simulink model "General_Stablised_Power_R2020a"  (R2020a)
settings: Solver=VariableStepAuto  StartTime=0.0  StopTime=10.0  FixedStep=1e-12  RelTol=1e-3
values from neighbouring files (symbols this model uses):
  Torque_Load = 1    [Parameters.m]
libraries: fl_lib x18, nesl_utility x18, ee_lib x13
settings Model: Creator=YXL1108  LastModifiedBy=YXL1108
settings SolverCC: ZeroCrossAlgorithm=Adaptive
settings DebuggingCC: IgnoredZcDiagnostic=none

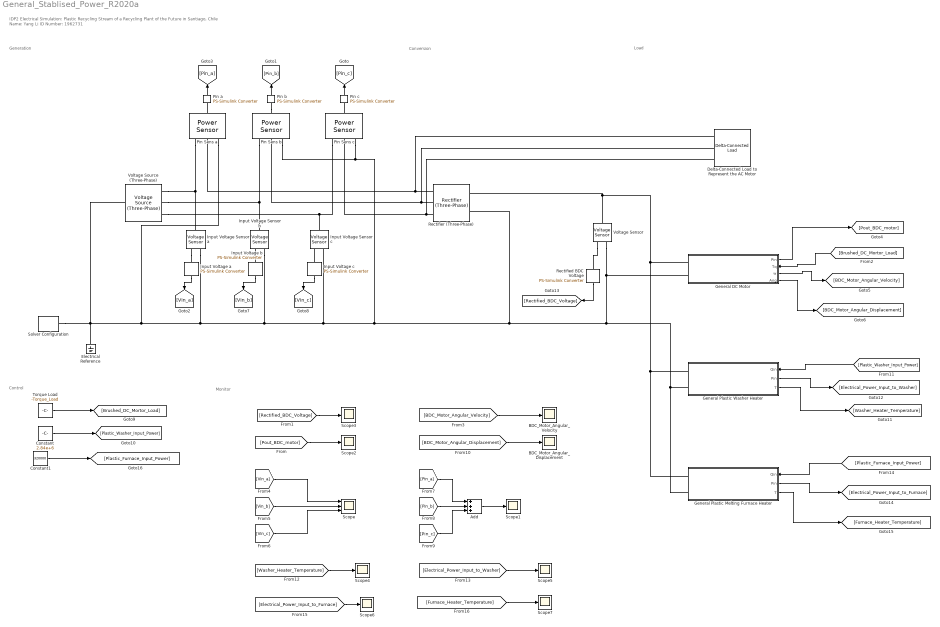
== system General_Stablised_Power_R2020a ==
  note: Control
  note: Load
  note: Conversion
  note: Monitor
  note: Generation
  note: IDP2 Electrical Simulation: Plastic Recycling Stream of a Recycling Plant of the Future in Santiago, Chile
      | Name: Yang Li
      | ID Number: 1962731
  Add : Sum  Inputs=+++
  BDC_Motor_Angular_Displacement : Scope
  BDC_Motor_Angular_Velocity : Scope
  Constant : Constant  Value=2.84e+6
  Constant1 : Constant  Value=320000
  Delta-Connected Load to Represent the AC Motor : ee_lib/Passive/RLC Assemblies/Delta-Connected Load  parameterization=2  component_structure=1  component_structure_PQ=4  R=1 Ohm  L=1e-3 H  C=1e-6 F  IL0=[0, 0, 0] A  VC0=[0, 0, 0] V  R_parasitic=1e-6 Ohm  G_parasitic=1e-6 1/Ohm  VRated=380 V  FRated=50 Hz  P=45 kW  Qpos=1e2 V*A  Qneg=-1e2 V*A  Vmag0=380 V  Vang0=0 deg  Freq0=50 Hz  R_parasitic_PQ=1e-6 Ohm  G_parasitic_PQ=1e-6 1/Ohm
      settings: SourceProductBaseCode=PS  InternalSimscapePortConfiguration="{\"Bottom\":[],\"Left\":[{\"id\":\"a\",\"label\":\"a\",\"type\":\"foundation.electrical.electrical\"},{\"id\":\"b\",\"label\":\"b\",\"type\":\"foundation.electrical.electrical\"},{\"id\":\"c\",\"label\":\"c\",\"type\":\"foundation.electrical.electrical\"}],\"Right\":[],\"Top\":[]}"
  Electrical Reference : fl_lib/Electrical/Electrical Elements/Electrical Reference
  General DC Motor : Subsystem
      settings: PortSchema="{\"entries\":[{\"content\":{\"sides\":[{\"content\":{\"connectorIds\":[\"LConn1\",\"LConn2\"]},\"type\":\"ConnectorPlacement.EquallySpacedRectSide\",\"uuid\":\"f4c4afdb-1f07-4496-beab-7bd7d7d73664\"},{\"content\":{\"connectorIds\":[\"Out1\",\"In1\",\"Out2\",\"Out3\"],\"side\":\"RIGHT\"},\"type\":\"ConnectorPlacement.EquallySpacedRectSide\",\"uuid\":\"dc37d443-6c2c-49b1-8221-5c741536e800\"},{\"content\":{\"connectorIds\":[],\"side\":\"TOP\"},\"type\":\"ConnectorPlacement.EquallySpacedRectSide\",\"uuid\":\"4c68adcc-5338-4c92-85dc-69672cfb0c08\"}]},\"type\":\"ConnectorPlacement.EquallySpacedConnector\",\"uuid\":\"b4ec0e54-21aa-4bd3-95d2-2023b489fb55\"}],\"packageUris\":[\"http://schema.mathworks.com/mf0/Connector/19700101\"],\"version\":\"1.0\"}"
  General Plastic Melting Furnace Heater : Subsystem
      settings: PortSchema="{\"entries\":[{\"content\":{\"sides\":[{\"content\":{\"connectorIds\":[\"LConn1\",\"LConn2\"]},\"type\":\"ConnectorPlacement.EquallySpacedRectSide\",\"uuid\":\"1fa59fc7-be06-49d0-a9b5-9f39dbd9f596\"},{\"content\":{\"connectorIds\":[\"In1\",\"Out1\",\"Out2\"],\"side\":\"RIGHT\"},\"type\":\"ConnectorPlacement.EquallySpacedRectSide\",\"uuid\":\"e02b180c-81d7-4bb9-9dca-301601ef73bf\"},{\"content\":{\"connectorIds\":[],\"side\":\"TOP\"},\"type\":\"ConnectorPlacement.EquallySpacedRectSide\",\"uuid\":\"9bedab00-a6ba-4834-a03a-1eed8c48595a\"}]},\"type\":\"ConnectorPlacement.EquallySpacedConnector\",\"uuid\":\"acdf9e6b-b46a-43ad-9e2b-2b45ab9d2f8b\"}],\"packageUris\":[\"http://schema.mathworks.com/mf0/Connector/19700101\"],\"version\":\"1.0\"}"
  General Plastic Washer Heater : Subsystem
      settings: PortSchema="{\"entries\":[{\"content\":{\"sides\":[{\"content\":{\"connectorIds\":[\"LConn1\",\"LConn2\"]},\"type\":\"ConnectorPlacement.EquallySpacedRectSide\",\"uuid\":\"1fa59fc7-be06-49d0-a9b5-9f39dbd9f596\"},{\"content\":{\"connectorIds\":[\"In1\",\"Out1\",\"Out2\"],\"side\":\"RIGHT\"},\"type\":\"ConnectorPlacement.EquallySpacedRectSide\",\"uuid\":\"e02b180c-81d7-4bb9-9dca-301601ef73bf\"},{\"content\":{\"connectorIds\":[],\"side\":\"TOP\"},\"type\":\"ConnectorPlacement.EquallySpacedRectSide\",\"uuid\":\"9bedab00-a6ba-4834-a03a-1eed8c48595a\"}]},\"type\":\"ConnectorPlacement.EquallySpacedConnector\",\"uuid\":\"acdf9e6b-b46a-43ad-9e2b-2b45ab9d2f8b\"}],\"packageUris\":[\"http://schema.mathworks.com/mf0/Connector/19700101\"],\"version\":\"1.0\"}"
  Input Voltage Sensor a : fl_lib/Electrical/Electrical Sensors/Voltage Sensor
  Input Voltage Sensor b : fl_lib/Electrical/Electrical Sensors/Voltage Sensor
  Input Voltage Sensor c : fl_lib/Electrical/Electrical Sensors/Voltage Sensor
  Input Voltage a : nesl_utility/PS-Simulink Converter  PhysicalDomain=network_engine_domain  SubClassName=ps_output  LeftPortType=input  RightPortType=output  PseudoPeriodic=off  Frequencies=[]  Unit=1  AffineConversion=off
  Input Voltage b : nesl_utility/PS-Simulink Converter  PhysicalDomain=network_engine_domain  SubClassName=ps_output  LeftPortType=input  RightPortType=output  PseudoPeriodic=off  Frequencies=[]  Unit=1  AffineConversion=off
  Input Voltage c : nesl_utility/PS-Simulink Converter  PhysicalDomain=network_engine_domain  SubClassName=ps_output  LeftPortType=input  RightPortType=output  PseudoPeriodic=off  Frequencies=[]  Unit=1  AffineConversion=off
  Pin Sens a : ee_lib/Sensors & Transducers/Power Sensor  measurement_type=1  averaging_period=1e-4 s
      settings: SourceProductBaseCode=PS
  Pin Sens b : ee_lib/Sensors & Transducers/Power Sensor  measurement_type=1  averaging_period=1e-4 s
      settings: SourceProductBaseCode=PS
  Pin Sens c : ee_lib/Sensors & Transducers/Power Sensor  measurement_type=1  averaging_period=1e-4 s
      settings: SourceProductBaseCode=PS
  Pin a : nesl_utility/PS-Simulink Converter  PhysicalDomain=network_engine_domain  SubClassName=ps_output  LeftPortType=input  RightPortType=output  PseudoPeriodic=off  Frequencies=[]  Unit=inherit  AffineConversion=off
  Pin b : nesl_utility/PS-Simulink Converter  PhysicalDomain=network_engine_domain  SubClassName=ps_output  LeftPortType=input  RightPortType=output  PseudoPeriodic=off  Frequencies=[]  Unit=inherit  AffineConversion=off
  Pin c : nesl_utility/PS-Simulink Converter  PhysicalDomain=network_engine_domain  SubClassName=ps_output  LeftPortType=input  RightPortType=output  PseudoPeriodic=off  Frequencies=[]  Unit=inherit  AffineConversion=off
  Rectified BDC Voltage : nesl_utility/PS-Simulink Converter  PhysicalDomain=network_engine_domain  SubClassName=ps_output  LeftPortType=input  RightPortType=output  PseudoPeriodic=off  Frequencies=[]  Unit=1  AffineConversion=off
  Rectifier (Three-Phase) : ee_lib/Semiconductors & Converters/Converters/Rectifier (Three-Phase)  model_dynamics=0  Vf=0.8 V  Ron=0.001 Ohm  Goff=1e-5 1/Ohm  C=50 nF  iRM=-235 A  iF=300 A  idot=-50 A/us  trr_param=1  trr_factor=3  trr=15 us  Qrr=1500 s*uA
      settings: SourceProductBaseCode=PS  InternalSimscapePortConfiguration="{\"Bottom\":[],\"Left\":[{\"id\":\"a\",\"label\":\"a\",\"type\":\"foundation.electrical.electrical\"},{\"id\":\"b\",\"label\":\"b\",\"type\":\"foundation.electrical.electrical\"},{\"id\":\"c\",\"label\":\"c\",\"type\":\"foundation.electrical.electrical\"}],\"Right\":[{\"id\":\"p\",\"label\":\"+\",\"type\":\"foundation.electrical.electrical\"},{\"id\":\"n\",\"label\":\"-\",\"type\":\"foundation.electrical.electrical\"}],\"Top\":[]}"
  Scope : Scope  NumInputPorts=3
  Scope{1..7} (7 alike) : Scope
  Solver Configuration : nesl_utility/Solver Configuration  PhysicalDomain=network_engine_domain  SubClassName=solver  LeftPortType=input  RightPortType=generic  Tones=[]  Harmonics=[]  SimulateNoise=off  Profile=off  UseLocalSampling=off  EnableSwitchedLinearOptims=on  FrequencyDomain=off  UseCCode=off  RelTol=0.001  AbsTol=1e-06  MinStep=1e-09  ToWorkspace=off  RevertToSquareIcSolve=off  NumHomotopyIterations=100  PhasorMode=off  PhasorModeNumHarmonics=1  DoDC=off  ResidualTolerance=1e-09  UseLocalSolver=off  LocalSolverChoice=NE_BACKWARD_EULER_ADVANCER  LocalSolverSampleTime=0.001  DoFixedCost=off  MaxNonlinIter=3  MaxModeIter=2  LinearAlgebra=auto  EquationFormulation=NE_TIME_EF  DelaysMemoryBudget=1024  AutomaticFiltering=on  FilteringTimeConstant=0.001  PartitionStorageMethod=AS_NEEDED  PartitionMemoryBudget=1024  PartitionMethod=ROBUST
  Torque Load : Constant  Value=-Torque_Load
  Voltage Source (Three-Phase) : ee_lib/Sources/Voltage Source (Three-Phase)  vline_rms=sqrt(3) * 380 / sqrt(2) V  shift=0 deg  freq=50 Hz  impedance_option=1  SShortCircuit=1e12 V*A  XR=15  R=0.01 Ohm  L=3.97e-4 H  G_parasitic=0 1/Ohm  harmonic_option=0  harmonic_orders=[5, 7, 11, 13]  harmonic_ratios=[.1, .1, .1, .1]  I_specify=off  I_priority=None  I=[ 0 0 0 ] A  I_nominal_specify=off  I_nominal_unit=A  I_nominal_value=1
      settings: SourceProductBaseCode=PS  InternalSimscapePortConfiguration="{\"Bottom\":[],\"Left\":[{\"id\":\"n\",\"label\":\"n\",\"type\":\"foundation.electrical.electrical\"}],\"Right\":[{\"id\":\"a\",\"label\":\"a\",\"type\":\"foundation.electrical.electrical\"},{\"id\":\"b\",\"label\":\"b\",\"type\":\"foundation.electrical.electrical\"},{\"id\":\"c\",\"label\":\"c\",\"type\":\"foundation.electrical.electrical\"}],\"Top\":[]}"
  Voltage Sensor : fl_lib/Electrical/Electrical Sensors/Voltage Sensor
  wires:
  Pin a/1 -> [Pin_a]
  Input Voltage b/1 -> [Vin_b]
  Input Voltage a/1 -> [Vin_a]
  Pin b/1 -> [Pin_b]
  Pin c/1 -> [Pin_c]
  Input Voltage c/1 -> [Vin_c]
  [Pin_b] -> Add/2
  Add/1 -> Scope1/1
  [Vin_a] -> Scope/1
  [Vin_b] -> Scope/2
  [Pin_a] -> Add/1
  [Vin_c] -> Scope/3
  [Pin_c] -> Add/3
  [Pout_BDC_motor] -> Scope2/1
  Rectified BDC Voltage/1 -> [Rectified_BDC_Voltage]
  [Rectified_BDC_Voltage] -> Scope3/1
  Torque Load/1 -> [Brushed_DC_Mortor_Load]
  [BDC_Motor_Angular_Displacement] -> BDC_Motor_Angular_Displacement/1
  [BDC_Motor_Angular_Velocity] -> BDC_Motor_Angular_Velocity/1
  [Brushed_DC_Mortor_Load] -> General DC Motor/1(Tq)
  General DC Motor/1(Pin) -> [Pout_BDC_motor]
  General DC Motor/2(w) -> [BDC_Motor_Angular_Velocity]
  General DC Motor/3(Ang) -> [BDC_Motor_Angular_Displacement]
  Constant/1 -> [Plastic_Washer_Input_Power]
  [Washer_Heater_Temperature] -> Scope4/1
  [Electrical_Power_Input_to_Washer] -> Scope5/1
  [Plastic_Washer_Input_Power] -> General Plastic Washer Heater/1(Qin)
  General Plastic Washer Heater/1(Pin) -> [Electrical_Power_Input_to_Washer]
  General Plastic Washer Heater/2(T) -> [Washer_Heater_Temperature]
  General Plastic Melting Furnace Heater/1(Pin) -> [Electrical_Power_Input_to_Furnace]
  General Plastic Melting Furnace Heater/2(T) -> [Furnace_Heater_Temperature]
  [Plastic_Furnace_Input_Power] -> General Plastic Melting Furnace Heater/1(Qin)
  Constant1/1 -> [Plastic_Furnace_Input_Power]
  [Electrical_Power_Input_to_Furnace] -> Scope6/1
  [Furnace_Heater_Temperature] -> Scope7/1
  connections:
  Voltage Source (Three-Phase)/RConn3 -- Pin Sens c/LConn1 -- Input Voltage Sensor c/LConn1
  Input Voltage Sensor b/RConn2 -- General Plastic Melting Furnace Heater/LConn2 -- General Plastic Washer Heater/LConn2 -- Voltage Sensor/RConn2 -- General DC Motor/LConn2 -- Rectifier (Three-Phase)/RConn2 -- Pin Sens c/LConn3 -- Pin Sens b/LConn3 -- Input Voltage Sensor c/RConn2 -- Pin Sens a/LConn3 -- Solver Configuration/RConn1 -- Electrical Reference/LConn1 -- Voltage Source (Three-Phase)/LConn1 -- Input Voltage Sensor a/RConn2
  Voltage Source (Three-Phase)/RConn2 -- Input Voltage Sensor b/LConn1 -- Pin Sens b/LConn1
  Pin Sens a/LConn1 -- Voltage Source (Three-Phase)/RConn1 -- Input Voltage Sensor a/LConn1
  Pin Sens a/RConn1 -- Pin a/LConn1
  Input Voltage c/LConn1 -- Input Voltage Sensor c/RConn1
  Input Voltage Sensor a/RConn1 -- Input Voltage a/LConn1
  Pin Sens c/RConn1 -- Pin c/LConn1
  Input Voltage b/LConn1 -- Input Voltage Sensor b/RConn1
  Pin b/LConn1 -- Pin Sens b/RConn1
  Voltage Sensor/LConn1 -- General Plastic Melting Furnace Heater/LConn1 -- General Plastic Washer Heater/LConn1 -- General DC Motor/LConn1 -- Rectifier (Three-Phase)/RConn1
  Voltage Sensor/RConn1 -- Rectified BDC Voltage/LConn1
  Rectifier (Three-Phase)/LConn1 -- Delta-Connected Load to Represent the AC Motor/LConn1 -- Pin Sens a/LConn2
  Rectifier (Three-Phase)/LConn2 -- Delta-Connected Load to Represent the AC Motor/LConn2 -- Pin Sens b/LConn2
  Rectifier (Three-Phase)/LConn3 -- Delta-Connected Load to Represent the AC Motor/LConn3 -- Pin Sens c/LConn2

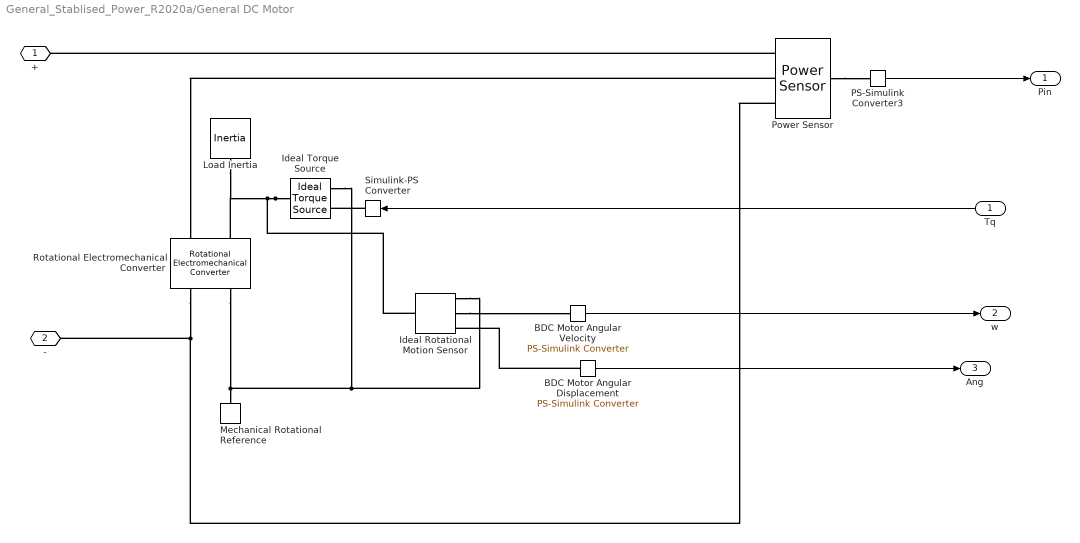
== system General_Stablised_Power_R2020a/General DC Motor ==
  Tq : Inport
  BDC Motor Angular Displacement : nesl_utility/PS-Simulink Converter  PhysicalDomain=network_engine_domain  SubClassName=ps_output  LeftPortType=input  RightPortType=output  PseudoPeriodic=off  Frequencies=[]  Unit=inherit  AffineConversion=off
      settings: SourceProductBaseCode=PW,SS
  BDC Motor Angular Velocity : nesl_utility/PS-Simulink Converter  PhysicalDomain=network_engine_domain  SubClassName=ps_output  LeftPortType=input  RightPortType=output  PseudoPeriodic=off  Frequencies=[]  Unit=inherit  AffineConversion=off
      settings: SourceProductBaseCode=PW,SS
  Ideal Rotational Motion Sensor : fl_lib/Mechanical/Mechanical Sensors/Ideal Rotational Motion Sensor  wrap_angle=simscape.enum.onoff.off  offset=0 rad
  Ideal Torque Source : fl_lib/Mechanical/Mechanical Sources/Ideal Torque Source
  Load Inertia : fl_lib/Mechanical/Rotational Elements/Inertia  inertia=0.01 kg*m^2  w_specify=off  w_priority=High  w=0 rad/s  w_nominal_specify=off  w_nominal_unit=rad/s  w_nominal_value=1  t_specify=off  t_priority=None  t=0 N*m  t_nominal_specify=off  t_nominal_unit=N*m  t_nominal_value=1
  Mechanical Rotational Reference : fl_lib/Mechanical/Rotational Elements/Mechanical Rotational Reference
  PS-Simulink Converter3 : nesl_utility/PS-Simulink Converter  PhysicalDomain=network_engine_domain  SubClassName=ps_output  LeftPortType=input  RightPortType=output  PseudoPeriodic=off  Frequencies=[]  Unit=inherit  AffineConversion=off
  Power Sensor : ee_lib/Sensors & Transducers/Power Sensor  measurement_type=1  averaging_period=1e-4 s
      settings: SourceProductBaseCode=PS
  Rotational Electromechanical Converter : fl_lib/Electrical/Electrical Elements/Rotational Electromechanical Converter  K=0.1 V/(rad/s)  i_specify=off  i_priority=None  i=0 A  i_nominal_specify=off  i_nominal_unit=A  i_nominal_value=1  v_specify=off  v_priority=None  v=0 V  v_nominal_specify=off  v_nominal_unit=V  v_nominal_value=1  t_specify=off  t_priority=None  t=0 N*m  t_nominal_specify=off  t_nominal_unit=N*m  t_nominal_value=1  w_specify=off  w_priority=None  w=0 rad/s  w_nominal_specify=off  w_nominal_unit=rad/s  w_nominal_value=1
  Simulink-PS Converter : nesl_utility/Simulink-PS Converter  PhysicalDomain=network_engine_domain  SubClassName=ps_input  LeftPortType=input  RightPortType=output  PseudoPeriodic=off  Frequencies=[]  NoiseDistribution=none  NoiseParameters=[]  Unit=1  AffineConversion=off  FilteringAndDerivatives=provide  SimscapeFilterOrder=1  InputFilterTimeConstant=0.001  UdotUserProvided=0
      settings: SourceProductBaseCode=PW,SS
  + : PMIOPort  Side=Left
  - : PMIOPort  Port=2  Side=Left
  Pin : Outport
  w : Outport  Port=2
  Ang : Outport  Port=3
  wires:
  BDC Motor Angular Velocity/1 -> w/1
  BDC Motor Angular Displacement/1 -> Ang/1
  PS-Simulink Converter3/1 -> Pin/1
  Tq/1 -> Simulink-PS Converter/1
  connections:
  Ideal Torque Source/LConn1 -- Rotational Electromechanical Converter/LConn2 -- Load Inertia/LConn1 -- Ideal Rotational Motion Sensor/LConn1
  Ideal Torque Source/RConn2 -- Ideal Rotational Motion Sensor/RConn1 -- Rotational Electromechanical Converter/RConn2 -- Mechanical Rotational Reference/LConn1
  Power Sensor/LConn2 -- Rotational Electromechanical Converter/LConn1
  Power Sensor/RConn1 -- PS-Simulink Converter3/LConn1
  Power Sensor/LConn3 -- Rotational Electromechanical Converter/RConn1 -- -/RConn1
  Simulink-PS Converter/RConn1 -- Ideal Torque Source/RConn1
  Ideal Rotational Motion Sensor/RConn2 -- BDC Motor Angular Velocity/LConn1
  BDC Motor Angular Displacement/LConn1 -- Ideal Rotational Motion Sensor/RConn3
  Power Sensor/LConn1 -- +/RConn1

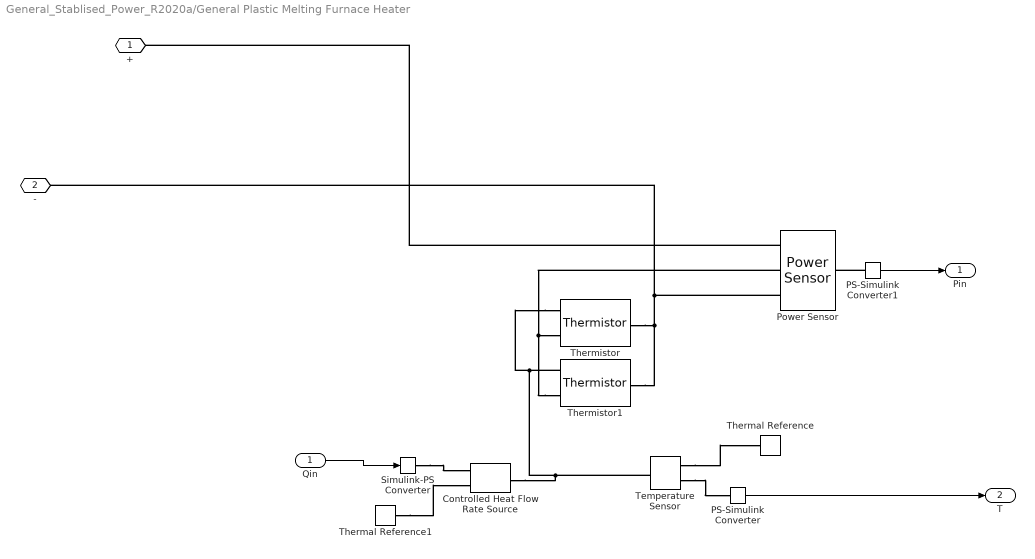
== system General_Stablised_Power_R2020a/General Plastic Melting Furnace Heater ==
  Qin : Inport
  Controlled Heat Flow Rate Source : fl_lib/Thermal/Thermal Sources/Controlled Heat Flow Rate Source
  PS-Simulink Converter : nesl_utility/PS-Simulink Converter  PhysicalDomain=network_engine_domain  SubClassName=ps_output  LeftPortType=input  RightPortType=output  PseudoPeriodic=off  Frequencies=[]  Unit=inherit  AffineConversion=off
  PS-Simulink Converter1 : nesl_utility/PS-Simulink Converter  PhysicalDomain=network_engine_domain  SubClassName=ps_output  LeftPortType=input  RightPortType=output  PseudoPeriodic=off  Frequencies=[]  Unit=inherit  AffineConversion=off
  Power Sensor : ee_lib/Sensors & Transducers/Power Sensor  measurement_type=1  averaging_period=1e-4 s
      settings: SourceProductBaseCode=PS
  Simulink-PS Converter : nesl_utility/Simulink-PS Converter  PhysicalDomain=network_engine_domain  SubClassName=ps_input  LeftPortType=input  RightPortType=output  PseudoPeriodic=off  Frequencies=[]  NoiseDistribution=none  NoiseParameters=[]  Unit=1  AffineConversion=off  FilteringAndDerivatives=provide  SimscapeFilterOrder=1  InputFilterTimeConstant=0.001  UdotUserProvided=0
  Temperature Sensor : fl_lib/Thermal/Thermal Sensors/Temperature Sensor
  Thermal Reference : fl_lib/Thermal/Thermal Elements/Thermal Reference
  Thermal Reference1 : fl_lib/Thermal/Thermal Elements/Thermal Reference
  Thermistor : ee_lib/Sensors & Transducers/Thermistor  R0=15000 Ohm  Bparam=3500 K  T0=293.15 K  tc=5.0 s  K_d=0.75e-3 W/K  T_specify=off  T_priority=High  T=298.15 K  T_nominal_specify=off  T_nominal_unit=K  T_nominal_value=1
      settings: SourceProductBaseCode=PS  InternalSimscapePortConfiguration="{\"Bottom\":[],\"Left\":[{\"id\":\"A\",\"label\":\"A\",\"type\":\"foundation.thermal.thermal\"},{\"id\":\"p\",\"label\":\"+\",\"type\":\"foundation.electrical.electrical\"}],\"Right\":[{\"id\":\"n\",\"label\":\"-\",\"type\":\"foundation.electrical.electrical\"}],\"Top\":[]}"
  Thermistor1 : ee_lib/Sensors & Transducers/Thermistor  R0=12000 Ohm  Bparam=3500 K  T0=293.15 K  tc=5.0 s  K_d=0.75e-3 W/K  T_specify=off  T_priority=High  T=298.15 K  T_nominal_specify=off  T_nominal_unit=K  T_nominal_value=1
      settings: SourceProductBaseCode=PS  InternalSimscapePortConfiguration="{\"Bottom\":[],\"Left\":[{\"id\":\"A\",\"label\":\"A\",\"type\":\"foundation.thermal.thermal\"},{\"id\":\"p\",\"label\":\"+\",\"type\":\"foundation.electrical.electrical\"}],\"Right\":[{\"id\":\"n\",\"label\":\"-\",\"type\":\"foundation.electrical.electrical\"}],\"Top\":[]}"
  + : PMIOPort  Side=Left
  - : PMIOPort  Port=2  Side=Left
  Pin : Outport
  T : Outport  Port=2
  wires:
  PS-Simulink Converter1/1 -> Pin/1
  Qin/1 -> Simulink-PS Converter/1
  PS-Simulink Converter/1 -> T/1
  connections:
  Power Sensor/LConn1 -- +/RConn1
  Thermal Reference1/LConn1 -- Controlled Heat Flow Rate Source/RConn2
  Temperature Sensor/RConn2 -- PS-Simulink Converter/LConn1
  PS-Simulink Converter1/LConn1 -- Power Sensor/RConn1
  -/RConn1 -- Power Sensor/LConn3 -- Thermistor/RConn1 -- Thermistor1/RConn1
  Thermistor1/LConn2 -- Thermistor/LConn2 -- Power Sensor/LConn2
  Thermistor/LConn1 -- Controlled Heat Flow Rate Source/LConn1 -- Temperature Sensor/LConn1 -- Thermistor1/LConn1
  Temperature Sensor/RConn1 -- Thermal Reference/LConn1
  Simulink-PS Converter/RConn1 -- Controlled Heat Flow Rate Source/RConn1

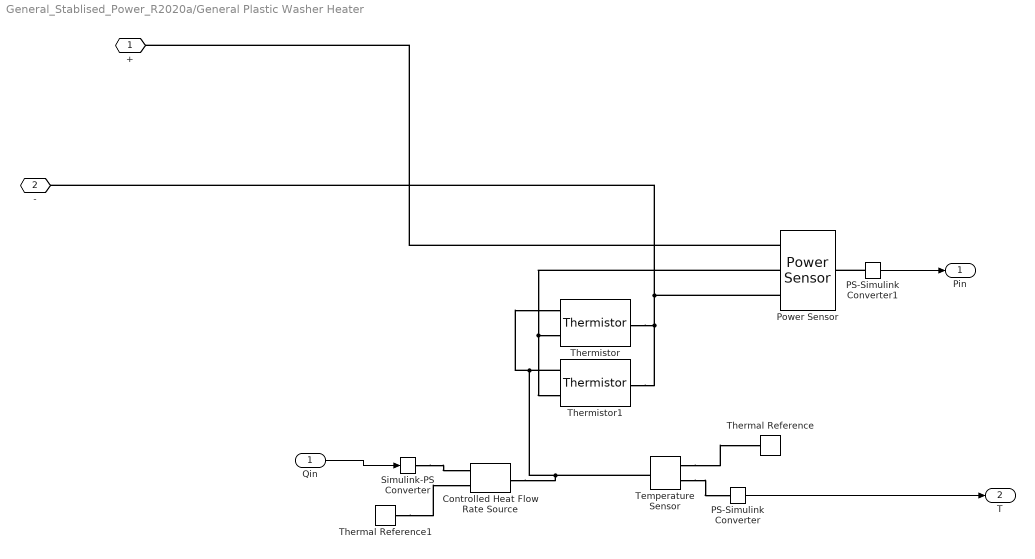
== system General_Stablised_Power_R2020a/General Plastic Washer Heater ==
  Qin : Inport
  Controlled Heat Flow Rate Source : fl_lib/Thermal/Thermal Sources/Controlled Heat Flow Rate Source
  PS-Simulink Converter : nesl_utility/PS-Simulink Converter  PhysicalDomain=network_engine_domain  SubClassName=ps_output  LeftPortType=input  RightPortType=output  PseudoPeriodic=off  Frequencies=[]  Unit=inherit  AffineConversion=off
  PS-Simulink Converter1 : nesl_utility/PS-Simulink Converter  PhysicalDomain=network_engine_domain  SubClassName=ps_output  LeftPortType=input  RightPortType=output  PseudoPeriodic=off  Frequencies=[]  Unit=inherit  AffineConversion=off
  Power Sensor : ee_lib/Sensors & Transducers/Power Sensor  measurement_type=1  averaging_period=1e-4 s
      settings: SourceProductBaseCode=PS
  Simulink-PS Converter : nesl_utility/Simulink-PS Converter  PhysicalDomain=network_engine_domain  SubClassName=ps_input  LeftPortType=input  RightPortType=output  PseudoPeriodic=off  Frequencies=[]  NoiseDistribution=none  NoiseParameters=[]  Unit=1  AffineConversion=off  FilteringAndDerivatives=provide  SimscapeFilterOrder=1  InputFilterTimeConstant=0.001  UdotUserProvided=0
  Temperature Sensor : fl_lib/Thermal/Thermal Sensors/Temperature Sensor
  Thermal Reference : fl_lib/Thermal/Thermal Elements/Thermal Reference
  Thermal Reference1 : fl_lib/Thermal/Thermal Elements/Thermal Reference
  Thermistor : ee_lib/Sensors & Transducers/Thermistor  R0=15000 Ohm  Bparam=3500 K  T0=293.15 K  tc=5.0 s  K_d=0.75e-3 W/K  T_specify=off  T_priority=High  T=298.15 K  T_nominal_specify=off  T_nominal_unit=K  T_nominal_value=1
      settings: SourceProductBaseCode=PS  InternalSimscapePortConfiguration="{\"Bottom\":[],\"Left\":[{\"id\":\"A\",\"label\":\"A\",\"type\":\"foundation.thermal.thermal\"},{\"id\":\"p\",\"label\":\"+\",\"type\":\"foundation.electrical.electrical\"}],\"Right\":[{\"id\":\"n\",\"label\":\"-\",\"type\":\"foundation.electrical.electrical\"}],\"Top\":[]}"
  Thermistor1 : ee_lib/Sensors & Transducers/Thermistor  R0=12000 Ohm  Bparam=3500 K  T0=293.15 K  tc=5.0 s  K_d=0.75e-3 W/K  T_specify=off  T_priority=High  T=298.15 K  T_nominal_specify=off  T_nominal_unit=K  T_nominal_value=1
      settings: SourceProductBaseCode=PS  InternalSimscapePortConfiguration="{\"Bottom\":[],\"Left\":[{\"id\":\"A\",\"label\":\"A\",\"type\":\"foundation.thermal.thermal\"},{\"id\":\"p\",\"label\":\"+\",\"type\":\"foundation.electrical.electrical\"}],\"Right\":[{\"id\":\"n\",\"label\":\"-\",\"type\":\"foundation.electrical.electrical\"}],\"Top\":[]}"
  + : PMIOPort  Side=Left
  - : PMIOPort  Port=2  Side=Left
  Pin : Outport
  T : Outport  Port=2
  wires:
  PS-Simulink Converter/1 -> T/1
  Qin/1 -> Simulink-PS Converter/1
  PS-Simulink Converter1/1 -> Pin/1
  connections:
  Simulink-PS Converter/RConn1 -- Controlled Heat Flow Rate Source/RConn1
  Temperature Sensor/RConn1 -- Thermal Reference/LConn1
  Controlled Heat Flow Rate Source/LConn1 -- Temperature Sensor/LConn1 -- Thermistor/LConn1 -- Thermistor1/LConn1
  Power Sensor/LConn2 -- Thermistor1/LConn2 -- Thermistor/LConn2
  Thermistor/RConn1 -- Thermistor1/RConn1 -- -/RConn1 -- Power Sensor/LConn3
  PS-Simulink Converter1/LConn1 -- Power Sensor/RConn1
  Temperature Sensor/RConn2 -- PS-Simulink Converter/LConn1
  Thermal Reference1/LConn1 -- Controlled Heat Flow Rate Source/RConn2
  Power Sensor/LConn1 -- +/RConn1
